simulink model "GoodWe_task"  (Simulink 3.00)
undefined symbols (not defined in the file): Byte, Double, F64, U8
libraries: mathlib x25, inoutlib x9, logiclib x6, arclib x6, matrixlib x5, paramlib x3, GoodWe_lib x2
settings Model: MaskType=REX sequence  MaskIconFrame=on  MaskIconOpaque=on  MaskIconRotate=none  MaskIconUnits=autoscale

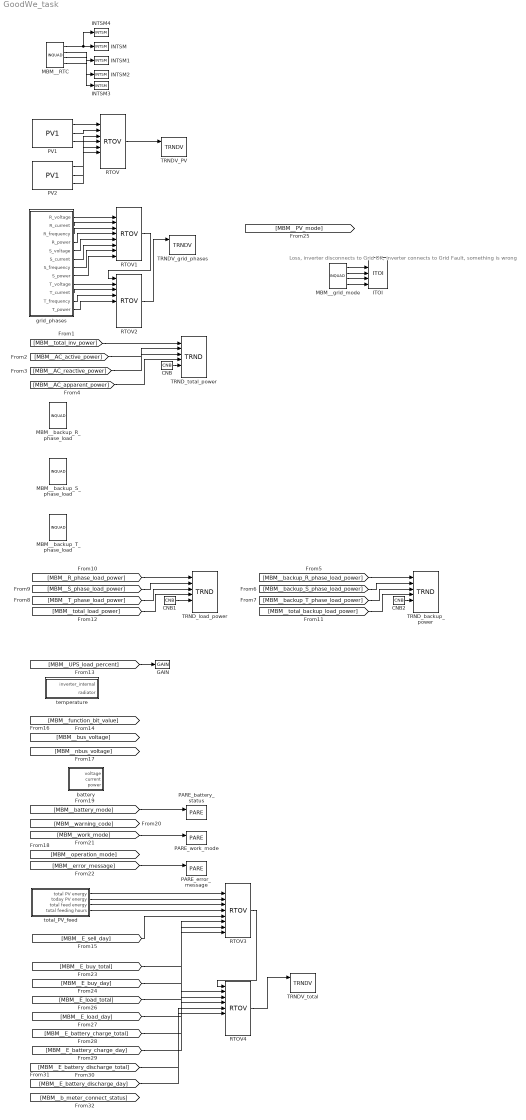
== system GoodWe_task ==
  note: Loss, inverter disconnects to Grid
      | OK, inverter connects to Grid
      | Fault, something is wrong
  CNB : mathlib/CNB  YCN=on
  CNB1 : mathlib/CNB  YCN=on
  CNB2 : mathlib/CNB  YCN=on
  GAIN : mathlib/GAIN  k=.01
  INTSM{,1..4} (5 alike) : logiclib/INTSM  shift=0  mask=-1  vtype=2: Byte (U8)
  ITOI : logiclib/ITOI  BINF=on  fktab=[1 2 4 0 0 0 0 0 0 0 0 0 0 0 0 0]
  MBM__RTC : inoutlib/INQUAD
  MBM__backup_R_phase_load : inoutlib/INQUAD
  MBM__backup_S_phase_load : inoutlib/INQUAD
  MBM__backup_T_phase_load : inoutlib/INQUAD
  MBM__grid_mode : inoutlib/INQUAD
  PARE_battery_status : paramlib/PARE  ipar=0: No battery, inverter disconnects to battery  pupstr=0: No battery, inverter disconnects to battery|1: Standby, no discharging and no charging|2: Discharging|3: Charging|4: Waiting for charge|5: Waiting for discharge\n  NUM=off  LIST=off  SATF=off
  PARE_error_message : paramlib/PARE  ipar=0: No error  pupstr=0: No error|1: GFCI Device Check Failure|2: AC HCT Check Failure|3: N/A|4: DCI Consistency Failure|5:GFCI Consistency Failure|6: N/A|7: GFCI Device Failure|8: Relay Device Failure|9: AC HCT Failure|10: Utility Loss|11: Ground I Failure|12: DC Bus High|13: Internal Fan Failure|14: Over Temperature|15: Utility Phase Failure|16: PV Over Voltage|17: External Fan Failure|18: Vac Failure|19: Isolation Failure|20: DC Injection High|21: Backup Overload|22: N/A|23: Fac Consistency Failure|24: Vac Consistency Failure|25: N/A|26: Relay Check Failure|27: N/A|28: Phase Angle Failure|29: DSP Communication Failure|30: Fac Failure|31: EEPROM R/W Failure|32: Internal Communication Failure  NUM=on  LIST=on  SATF=off
  PARE_work_mode : paramlib/PARE  ipar=0: No battery, inverter disconnects to battery  pupstr=0: Wait - Cut of all the connection to inverter|1: On-Grid - PV inputs to inverter, inverter outputs to grid|2: Off-Grid - PV inputs to inverter (first), battery inputs to inverter (second), inverter work as AC source|3: Fault|4: Flash - Inverter upgrade|5: Check - Power on self-check of inverter\n  NUM=off  LIST=off  SATF=off
  PV1 : GoodWe_lib/PV1  id=1
  PV2 : GoodWe_lib/PV1  id=2
  RTOV : matrixlib/RTOV  nmax=8  offset=0  n=8  etype=8: Double (F64)
  RTOV1 : matrixlib/RTOV  nmax=12  offset=0  n=8  etype=8: Double (F64)
  RTOV2 : matrixlib/RTOV  nmax=12  offset=8  n=4  etype=8: Double (F64)
  RTOV3 : matrixlib/RTOV  nmax=16  offset=0  n=8  etype=8: Double (F64)
  RTOV4 : matrixlib/RTOV  nmax=16  offset=8  n=8  etype=8: Double (F64)
  TRNDV_PV : arclib/TRNDV  n=6  l=10000  btype=8: Double (F64)  pfac=1  afac=1  arc=1  id=1  Title=PV State  timesrc=1: CORETIMER  SigNames=PV1 voltage\nPV1 current\nPV1 power\nPV2 voltage\nPV2 current\nPV2 power  ViewConfig="{\"View\":{\"Data\":{\"History\":30.517578125,\"XAxisTimeFormat\":66},\"PropertiesModel\":[{\"Id\":0,\"Items\":[{\"Color\":\"#000099\",\"Id\":0,\"IsActive\":true,\"LineWidth\":2,\"Name\":\"PV1 voltage\",\"SceneNumber\":25},{\"Color\":\"#669900\",\"Id\":1,\"IsActive\":true,\"LineWidth\":2,\"Name\":\"PV1 current\",\"SceneNumber\":26},{\"Color\":\"#ff0000\",\"Id\":2,\"IsActive\":true,\"LineWidth\":2,\"Name\":\"PV1 power\",\"SceneNumber\":27},{\"Color\":\"#9966cc\",\"Id\":3,\"IsActive\":true,\"LineWidth\":2,\"Name\":\"PV2 voltage\",\"SceneNumber\":25},{\"Color\":\"#339999\",\"Id\":4,\"IsActive\":true,\"LineWidth\":2,\"Name\":\"PV2 current\",\"SceneNumber\":26},{\"Color\":\"#996600\",\"Id\":5,\"IsActive\":true,\"LineWidth\":2,\"Name\":\"PV2 power\",\"SceneNumber\":27}]}],\"Scenes\":[{\"Id\":25},{\"Id\":26},{\"Id\":27}],\"sync\":false}}"
  TRNDV_grid_phases : arclib/TRNDV  n=12  l=10000  btype=8: Double (F64)  pfac=1  afac=1  arc=1  id=2  Title=Trend Title  timesrc=1: CORETIMER  ViewConfig="{\"View\":{\"Data\":{\"History\":439.80465111040024,\"XAxisTimeFormat\":66},\"PropertiesModel\":[{\"Id\":0,\"Items\":[{\"Color\":\"#000099\",\"Id\":0,\"IsActive\":true,\"LineWidth\":2,\"Name\":\"L1 voltage\",\"SceneNumber\":31},{\"Color\":\"#669900\",\"Id\":1,\"IsActive\":true,\"LineWidth\":2,\"Name\":\"L1 current\",\"SceneNumber\":32},{\"Color\":\"#ff0000\",\"Id\":2,\"IsActive\":true,\"LineWidth\":2,\"Name\":\"L1 frequency\",\"SceneNumber\":33},{\"Color\":\"#9966cc\",\"Id\":3,\"IsActive\":true,\"LineWidth\":2,\"Name\":\"L1 power\",\"SceneNumber\":34},{\"Color\":\"#339999\",\"Id\":4,\"IsActive\":true,\"LineWidth\":2,\"Name\":\"L2 voltage\",\"SceneNumber\":31},{\"Color\":\"#996600\",\"Id\":5,\"IsActive\":true,\"LineWidth\":2,\"Name\":\"L2 current\",\"SceneNumber\":32},{\"Color\":\"#ff6666\",\"Id\":6,\"IsActive\":true,\"LineWidth\":2,\"Name\":\"L2 frequency\",\"SceneNumber\":33},{\"Color\":\"#006600\",\"Id\":7,\"IsActive\":true,\"LineWidth\":2,\"Name\":\"L2 power\",\"SceneNumber\":34},{\"Color\":\"#990066\",\"Id\":8,\"IsActive\":true,\"LineWidth\":2,\"Name\":\"L3 voltage\",\"SceneNumber\":31},{\"Color\":\"#cc9900\",\"Id\":9,\"IsActive\":true,\"LineWidth\":2,\"Name\":\"L3 current\",\"SceneNumber\":32},{\"Color\":\"#330066\",\"Id\":10,\"IsActive\":true,\"LineWidth\":2,\"Name\":\"L3 frequency\",\"SceneNumber\":33},{\"Color\":\"#ff6600\",\"Id\":11,\"IsActive\":true,\"LineWidth\":2,\"Name\":\"L3 power\",\"SceneNumber\":34}]}],\"Scenes\":[{\"Id\":31},{\"Id\":32},{\"Id\":33},{\"Id\":34}],\"sync\":false}}"
  TRNDV_total : arclib/TRNDV  n=12  l=10000  btype=8: Double (F64)  pfac=1  afac=1  arc=1  id=4  Title=Trend Title  timesrc=1: CORETIMER  ViewConfig="{\"View\":{\"Data\":{\"History\":439.80465111040024,\"XAxisTimeFormat\":66},\"PropertiesModel\":[{\"Id\":0,\"Items\":[{\"Color\":\"#000099\",\"Id\":0,\"IsActive\":true,\"LineWidth\":2,\"Name\":\"signal 1\",\"SceneNumber\":16},{\"Color\":\"#669900\",\"Id\":1,\"IsActive\":true,\"LineWidth\":2,\"SceneNumber\":17},{\"Color\":\"#ff0000\",\"Id\":2,\"IsActive\":true,\"LineWidth\":2,\"SceneNumber\":18},{\"Color\":\"#9966cc\",\"Id\":3,\"IsActive\":true,\"LineWidth\":2,\"SceneNumber\":19},{\"Color\":\"#339999\",\"Id\":4,\"IsActive\":true,\"LineWidth\":2,\"SceneNumber\":16},{\"Color\":\"#996600\",\"Id\":5,\"IsActive\":true,\"LineWidth\":2,\"SceneNumber\":17},{\"Color\":\"#ff6666\",\"Id\":6,\"IsActive\":true,\"LineWidth\":2,\"SceneNumber\":18},{\"Color\":\"#006600\",\"Id\":7,\"IsActive\":true,\"LineWidth\":2,\"SceneNumber\":19},{\"Color\":\"#990066\",\"Id\":8,\"IsActive\":true,\"LineWidth\":2,\"SceneNumber\":16},{\"Color\":\"#cc9900\",\"Id\":9,\"IsActive\":true,\"LineWidth\":2,\"SceneNumber\":17},{\"Color\":\"#330066\",\"Id\":10,\"IsActive\":true,\"LineWidth\":2,\"SceneNumber\":18},{\"Color\":\"#ff6600\",\"Id\":11,\"IsActive\":true,\"LineWidth\":2,\"SceneNumber\":19}]}],\"Scenes\":[{\"Id\":16},{\"Id\":17},{\"Id\":18},{\"Id\":19}],\"sync\":false}}"
  TRND_backup_power : arclib/TRND  n=4  l=10000  btype=8: Double (F64)  ptype1=1: Store  ptype2=1: Store  ptype3=1: Store  ptype4=1: Store  pfac=1  afac=1  arc=1  id=6  Title=Backup power  timesrc=1: CORETIMER  ViewConfig="{\"View\":{\"Data\":{\"History\":30.22314549036578,\"XAxisTimeFormat\":66},\"PropertiesModel\":[{\"Id\":0,\"Items\":[{\"Color\":\"#000099\",\"Id\":0,\"IsActive\":true,\"LineWidth\":2,\"Name\":\"L1\",\"SceneNumber\":39},{\"Color\":\"#669900\",\"Id\":1,\"IsActive\":true,\"LineWidth\":2,\"Name\":\"L2\",\"SceneNumber\":39},{\"Color\":\"#ff0000\",\"Id\":2,\"IsActive\":true,\"LineWidth\":2,\"Name\":\"L3\",\"SceneNumber\":39},{\"Color\":\"#9966cc\",\"Id\":3,\"IsActive\":true,\"LineWidth\":2,\"Name\":\"total\",\"SceneNumber\":39}]}],\"Scenes\":[{\"Id\":39}],\"sync\":false}}"
  TRND_load_power : arclib/TRND  n=4  l=10000  btype=8: Double (F64)  ptype1=1: Store  ptype2=1: Store  ptype3=1: Store  ptype4=1: Store  pfac=1  afac=1  arc=1  id=5  Title=Load power  timesrc=1: CORETIMER  ViewConfig="{\"View\":{\"Data\":{\"History\":30.22314549036578,\"XAxisTimeFormat\":66},\"PropertiesModel\":[{\"Id\":0,\"Items\":[{\"Color\":\"#000099\",\"Id\":0,\"IsActive\":true,\"LineWidth\":2,\"Name\":\"L1\",\"SceneNumber\":39},{\"Color\":\"#669900\",\"Id\":1,\"IsActive\":true,\"LineWidth\":2,\"Name\":\"L2\",\"SceneNumber\":39},{\"Color\":\"#ff0000\",\"Id\":2,\"IsActive\":true,\"LineWidth\":2,\"Name\":\"L3\",\"SceneNumber\":39},{\"Color\":\"#9966cc\",\"Id\":3,\"IsActive\":true,\"LineWidth\":2,\"Name\":\"total\",\"SceneNumber\":39}]}],\"Scenes\":[{\"Id\":39}],\"sync\":false}}"
  TRND_total_power : arclib/TRND  n=4  l=10000  btype=8: Double (F64)  ptype1=1: Store  ptype2=1: Store  ptype3=1: Store  ptype4=1: Store  pfac=1  afac=1  arc=1  id=3  Title=Trend Title  timesrc=1: CORETIMER  ViewConfig="{\"View\":{\"Data\":{\"History\":2097.1520000000014,\"XAxisTimeFormat\":66},\"PropertiesModel\":[{\"Id\":0,\"Items\":[{\"Color\":\"#000099\",\"Id\":0,\"IsActive\":true,\"LineWidth\":2,\"Name\":\"total inverter power\",\"SceneNumber\":35},{\"Color\":\"#669900\",\"Id\":1,\"IsActive\":true,\"LineWidth\":2,\"Name\":\"AC active power\",\"SceneNumber\":35},{\"Color\":\"#ff0000\",\"Id\":2,\"IsActive\":true,\"LineWidth\":2,\"SceneNumber\":35},{\"Color\":\"#9966cc\",\"Id\":3,\"IsActive\":true,\"LineWidth\":2,\"SceneNumber\":35}]}],\"Scenes\":[{\"Id\":35}],\"sync\":false}}"
  battery : Subsystem
      mask Type: REX sequence
  grid_phases : Subsystem
      mask Type: REX sequence
  temperature : Subsystem
      mask Type: REX sequence
  total_PV_feed : Subsystem
      mask Type: REX sequence
  wires:
  CNB/1 -> TRND_total_power/5
  CNB1/1 -> TRND_load_power/5
  CNB2/1 -> TRND_backup_power/5
  [MBM__total_inv_power] -> TRND_total_power/1
  [MBM__R_phase_load_power] -> TRND_load_power/1
  [MBM__total_backup_load_power] -> TRND_backup_power/4
  [MBM__total_load_power] -> TRND_load_power/4
  [MBM__UPS_load_percent] -> GAIN/1
  [MBM__E_sell_day] -> RTOV3/6
  [MBM__battery_mode] -> PARE_battery_status/1
  [MBM__AC_active_power] -> TRND_total_power/2
  [MBM__work_mode] -> PARE_work_mode/1
  [MBM__error_message] -> PARE_error_message/1
  [MBM__E_buy_total] -> RTOV3/7
  [MBM__E_buy_day] -> RTOV3/8
  [MBM__E_load_total] -> RTOV3/9
  [MBM__E_load_day] -> RTOV4/2
  [MBM__E_battery_charge_total] -> RTOV4/3
  [MBM__E_battery_charge_day] -> RTOV4/4
  [MBM__AC_reactive_power] -> TRND_total_power/3
  [MBM__E_battery_discharge_total] -> RTOV4/5
  [MBM__E_battery_discharge_day] -> RTOV4/6
  [MBM__AC_apparent_power] -> TRND_total_power/4
  [MBM__backup_R_phase_load_power] -> TRND_backup_power/1
  [MBM__backup_S_phase_load_power] -> TRND_backup_power/2
  [MBM__backup_T_phase_load_power] -> TRND_backup_power/3
  [MBM__T_phase_load_power] -> TRND_load_power/3
  [MBM__S_phase_load_power] -> TRND_load_power/2
  MBM__RTC/1 -> INTSM/1, INTSM4/1
  MBM__RTC/2 -> INTSM1/1
  MBM__RTC/3 -> INTSM2/1
  MBM__RTC/4 -> INTSM3/1
  MBM__grid_mode/1 -> ITOI/2
  MBM__grid_mode/2 -> ITOI/3
  MBM__grid_mode/3 -> ITOI/4
  MBM__grid_mode/4 -> ITOI/5
  PV1/1 -> RTOV/2
  PV1/2 -> RTOV/3
  PV1/3 -> RTOV/4
  PV2/1 -> RTOV/5
  PV2/2 -> RTOV/6
  PV2/3 -> RTOV/7
  RTOV/1 -> TRNDV_PV/1
  RTOV1/1 -> RTOV2/1
  RTOV2/1 -> TRNDV_grid_phases/1
  RTOV3/1 -> RTOV4/1
  RTOV4/1 -> TRNDV_total/1
  grid_phases/1(R_voltage) -> RTOV1/2
  grid_phases/2(R_current) -> RTOV1/3
  grid_phases/3(R_frequency) -> RTOV1/4
  grid_phases/4(R_power) -> RTOV1/5
  grid_phases/5(S_voltage) -> RTOV1/6
  grid_phases/6(S_current) -> RTOV1/7
  grid_phases/7(S_frequency) -> RTOV1/8
  grid_phases/8(S_power) -> RTOV1/9
  grid_phases/9(T_voltage) -> RTOV2/2
  grid_phases/10(T_current) -> RTOV2/3
  grid_phases/11(T_frequency) -> RTOV2/4
  grid_phases/12(T_power) -> RTOV2/5
  total_PV_feed/1(total PV energy) -> RTOV3/2
  total_PV_feed/2(today PV energy) -> RTOV3/3
  total_PV_feed/3(total feed energy) -> RTOV3/4
  total_PV_feed/4(total feeding hours) -> RTOV3/5

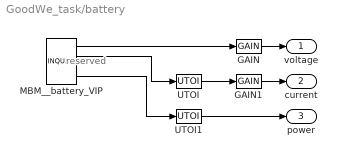
== system GoodWe_task/battery ==
  note: reserved
  GAIN : mathlib/GAIN  k=.1
  GAIN1 : mathlib/GAIN  k=.1
  MBM__battery_VIP : inoutlib/INQUAD
  UTOI : mathlib/UTOI  bits=16  SWAP=off
  UTOI1 : mathlib/UTOI  bits=16  SWAP=off
  voltage : Outport  Port=1  OutDataTypeStr=Inherit: auto
  current : Outport  Port=2  OutDataTypeStr=Inherit: auto
  power : Outport  Port=3  OutDataTypeStr=Inherit: auto
  wires:
  GAIN/1 -> voltage/1
  GAIN1/1 -> current/1
  MBM__battery_VIP/1 -> GAIN/1
  MBM__battery_VIP/2 -> UTOI/1
  MBM__battery_VIP/4 -> UTOI1/1
  UTOI/1 -> GAIN1/1
  UTOI1/1 -> power/1

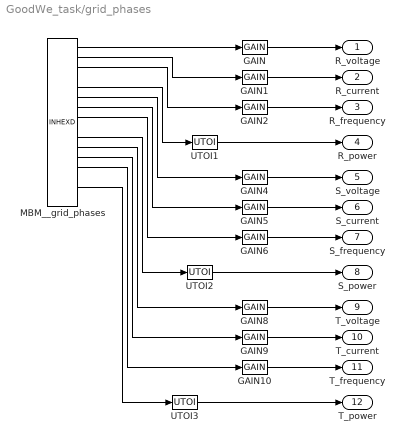
== system GoodWe_task/grid_phases ==
  GAIN{,1,4..5,8..9} (6 alike) : mathlib/GAIN  k=0.1
  GAIN10 : mathlib/GAIN  k=0.01
  GAIN2 : mathlib/GAIN  k=0.01
  GAIN6 : mathlib/GAIN  k=0.01
  MBM__grid_phases : inoutlib/INHEXD
  UTOI1 : mathlib/UTOI  bits=16  SWAP=off
  UTOI2 : mathlib/UTOI  bits=16  SWAP=off
  UTOI3 : mathlib/UTOI  bits=16  SWAP=off
  R_voltage : Outport  Port=1  OutDataTypeStr=Inherit: auto
  R_current : Outport  Port=2  OutDataTypeStr=Inherit: auto
  R_frequency : Outport  Port=3  OutDataTypeStr=Inherit: auto
  R_power : Outport  Port=4  OutDataTypeStr=Inherit: auto
  S_voltage : Outport  Port=5  OutDataTypeStr=Inherit: auto
  S_current : Outport  Port=6  OutDataTypeStr=Inherit: auto
  S_frequency : Outport  Port=7  OutDataTypeStr=Inherit: auto
  S_power : Outport  Port=8  OutDataTypeStr=Inherit: auto
  T_voltage : Outport  Port=9  OutDataTypeStr=Inherit: auto
  T_current : Outport  Port=10  OutDataTypeStr=Inherit: auto
  T_frequency : Outport  Port=11  OutDataTypeStr=Inherit: auto
  T_power : Outport  Port=12  OutDataTypeStr=Inherit: auto
  wires:
  GAIN/1 -> R_voltage/1
  GAIN1/1 -> R_current/1
  GAIN10/1 -> T_frequency/1
  GAIN2/1 -> R_frequency/1
  GAIN4/1 -> S_voltage/1
  GAIN5/1 -> S_current/1
  GAIN6/1 -> S_frequency/1
  GAIN8/1 -> T_voltage/1
  GAIN9/1 -> T_current/1
  MBM__grid_phases/1 -> GAIN/1
  MBM__grid_phases/2 -> GAIN1/1
  MBM__grid_phases/3 -> GAIN2/1
  MBM__grid_phases/5 -> UTOI1/1
  MBM__grid_phases/6 -> GAIN4/1
  MBM__grid_phases/7 -> GAIN5/1
  MBM__grid_phases/8 -> GAIN6/1
  MBM__grid_phases/10 -> UTOI2/1
  MBM__grid_phases/11 -> GAIN8/1
  MBM__grid_phases/12 -> GAIN9/1
  MBM__grid_phases/13 -> GAIN10/1
  MBM__grid_phases/15 -> UTOI3/1
  UTOI1/1 -> R_power/1
  UTOI2/1 -> S_power/1
  UTOI3/1 -> T_power/1

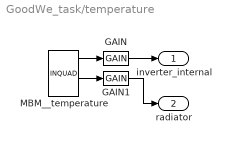
== system GoodWe_task/temperature ==
  GAIN : mathlib/GAIN  k=.1
  GAIN1 : mathlib/GAIN  k=.1
  MBM__temperature : inoutlib/INQUAD
  inverter_internal : Outport  Port=1  OutDataTypeStr=Inherit: auto
  radiator : Outport  Port=2  OutDataTypeStr=Inherit: auto
  wires:
  GAIN/1 -> inverter_internal/1
  GAIN1/1 -> radiator/1
  MBM__temperature/1 -> GAIN/1
  MBM__temperature/3 -> GAIN1/1

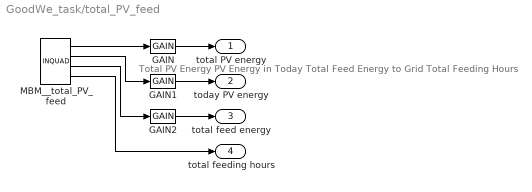
== system GoodWe_task/total_PV_feed ==
  note: Total PV Energy
      | PV Energy in Today
      | Total Feed Energy to Grid
      | Total Feeding Hours
  GAIN : mathlib/GAIN  k=.1
  GAIN1 : mathlib/GAIN  k=.1
  GAIN2 : mathlib/GAIN  k=.1
  MBM__total_PV_feed : inoutlib/INQUAD
  total PV energy : Outport  Port=1  OutDataTypeStr=Inherit: auto
  today PV energy : Outport  Port=2  OutDataTypeStr=Inherit: auto
  total feed energy : Outport  Port=3  OutDataTypeStr=Inherit: auto
  total feeding hours : Outport  Port=4  OutDataTypeStr=Inherit: auto
  wires:
  GAIN/1 -> total PV energy/1
  GAIN1/1 -> today PV energy/1
  GAIN2/1 -> total feed energy/1
  MBM__total_PV_feed/1 -> GAIN/1
  MBM__total_PV_feed/2 -> GAIN1/1
  MBM__total_PV_feed/3 -> GAIN2/1
  MBM__total_PV_feed/4 -> total feeding hours/1
